simulink model "PWM_IM"  (Simulink 7.3)
settings: Solver=ode45  StartTime=0.0  StopTime=.5  RelTol=1e-3
libraries: powerlib x9
settings Model: Creator=Debmalya Mukherjee  LastModifiedBy=Debmalya Mukherjee

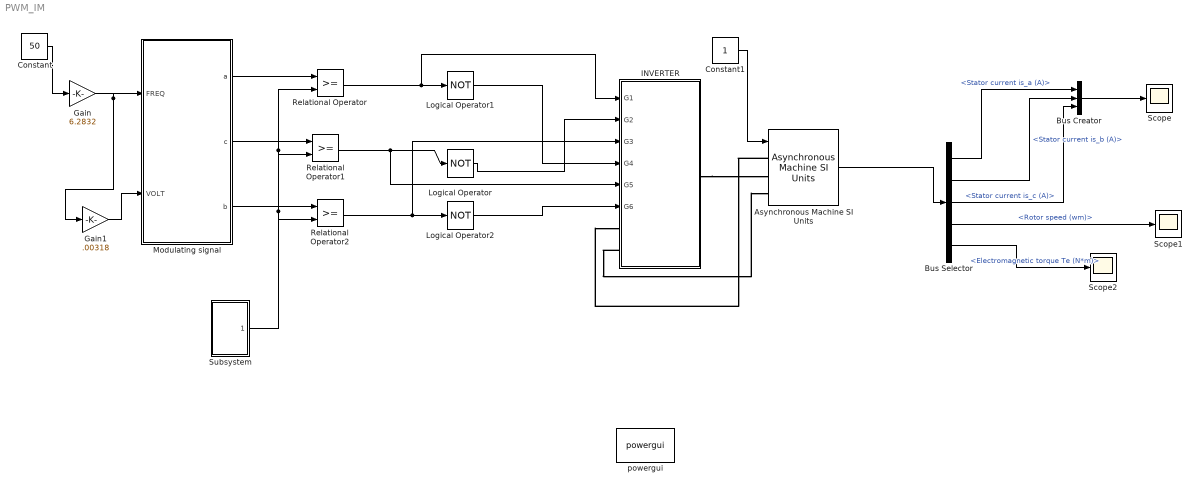
== system PWM_IM ==
  Asynchronous Machine SI Units : powerlib/Machines/Asynchronous Machine SI Units  DialogController=POWERSYS.PowerSysDialog  SystemSampleTime=-1  PresetModel=No  MechanicalLoad=Torque Tm  ShowDetailedParameters=on  RotorType=Squirrel-cage  ReferenceFrame=Rotor  NominalParameters=[10422.6 415 50 ]  Stator=[1.09 .006]  Rotor=[1.09 .006]  Lm=.072  Mechanical=[.1 .03 2]  PolePairs=2  InitialConditions=[1 0 0 0 0 0 0 0]  Units=SI  LoadFlowParameters=1492000  SimulateSaturation=off  Saturation=[14.03593122, 27.81365428, 53.79336849, 72.68890987, 97.98006896, 148.6815601, 215.7428561, 302.9841135, 428.7778367 ; 230, 322, 414, 460, 506, 552, 598, 644, 690]  TsPowergui=0  TsBlock=-1  IterativeModel=Forward Euler
  Bus Creator : BusCreator  Inputs=3
  Bus Selector : BusSelector  OutputSignals=Stator measurements.Stator current is_a (A),Stator measurements.Stator current is_b (A),Stator measurements.Stator current is_c (A),Mechanical.Rotor speed (wm),Mechanical.Electromagnetic torque Te (N*m)
  Constant : Constant  Value=50  OutDataType=fixdt(1, 16)  OutScaling=2^0
  Constant1 : Constant  OutDataType=fixdt(1, 16)  OutScaling=2^0
  Gain : Gain  Gain=6.2832  ParameterDataType=fixdt(1, 16)  ParameterScaling=2^0  OutDataType=fixdt(1, 16)  OutScaling=2^0
  Gain1 : Gain  Gain=.00318  ParameterDataType=fixdt(1, 16)  ParameterScaling=2^0  OutDataType=fixdt(1, 16)  OutScaling=2^0
  INVERTER : Subsystem
  Logical Operator : Logic  Operator=NOT  AllPortsSameDT=off  OutDataTypeMode=boolean  LogicDataType=fixdt(0, 8)  OutDataTypeStr=boolean
  Logical Operator1 : Logic  Operator=NOT  AllPortsSameDT=off  OutDataTypeMode=boolean  LogicDataType=fixdt(0, 8)  OutDataTypeStr=boolean
  Logical Operator2 : Logic  Operator=NOT  AllPortsSameDT=off  OutDataTypeMode=boolean  LogicDataType=fixdt(0, 8)  OutDataTypeStr=boolean
  Modulating signal : Subsystem
  Relational Operator : RelationalOperator  LogicOutDataTypeMode=boolean  LogicDataType=fixdt(0, 8)  OutDataTypeStr=boolean
  Relational Operator1 : RelationalOperator  LogicOutDataTypeMode=boolean  LogicDataType=fixdt(0, 8)  OutDataTypeStr=boolean
  Relational Operator2 : RelationalOperator  LogicOutDataTypeMode=boolean  LogicDataType=fixdt(0, 8)  OutDataTypeStr=boolean
  Scope : Scope
      settings: TimeRange=0.0291187739463602  YMin=-100  YMax=150
  Scope1 : Scope
  Scope2 : Scope
      settings: SaveName=ScopeData2
  Subsystem : Subsystem
  powergui : powerlib/powergui  Priority=1  SystemSampleTime=-1  SimulationMode=Continuous  SampleTime=50e-6  frequency=60  SPID=off  DisableSnubberDevices=off  DisableRonSwitches=off  DisableVfSwitches=off  SwTol=0  Interpol=off  frequencyindice=50  echomessages=off  HookPort=off  DisplayEquations=off  FunctionMessages=off  EnableUseOfTLC=off  x0status=blocks  RestoreLinks=warning  Frange=[0:2:500]  Ylog=off  Xlog=on  ShowGrid=off  save=off  variable=ZData  ZoomFFT=on  StartTime=0.0  cycles=1  DisplayStyle=1  fundamental=60  FreqAxis=off  MaxFrequency=1000  frequencyindicesteady=1  RmsSteady=1  display=off  Ts=0  methode=off
  wires:
  Constant/1 -> Gain/1
  Gain/1 -> Gain1/1, Modulating signal/1(FREQ)
  Gain1/1 -> Modulating signal/2(VOLT)
  Constant1/1 -> Asynchronous Machine SI Units/1
  Subsystem/1(Carrier) -> Relational Operator2/2, Relational Operator/2, Relational Operator1/2
  Modulating signal/1(a) -> Relational Operator/1
  Modulating signal/2(c) -> Relational Operator1/1
  Modulating signal/3(b) -> Relational Operator2/1
  Relational Operator/1 -> Logical Operator1/1, INVERTER/1(G1)
  Logical Operator1/1 -> INVERTER/4(G4)
  Relational Operator2/1 -> Logical Operator2/1, INVERTER/3(G3)
  Logical Operator2/1 -> INVERTER/6(G6)
  Relational Operator1/1 -> Logical Operator/1, INVERTER/5(G5)
  Logical Operator/1 -> INVERTER/2(G2)
  Asynchronous Machine SI Units/1 -> Bus Selector/1
  Bus Selector/1 -> Bus Creator/1  "<Stator current is_a (A)>"
  Bus Selector/2 -> Bus Creator/2  "<Stator current is_b (A)>"
  Bus Selector/3 -> Bus Creator/3  "<Stator current is_c (A)>"
  Bus Creator/1 -> Scope/1
  Bus Selector/4 -> Scope1/1  "<Rotor speed (wm)>"
  Bus Selector/5 -> Scope2/1  "<Electromagnetic torque Te (N*m)>"
  connections:
  INVERTER/RConn1 -- Asynchronous Machine SI Units/LConn2
  INVERTER/LConn2 -- Asynchronous Machine SI Units/LConn3
  Asynchronous Machine SI Units/LConn1 -- INVERTER/LConn1

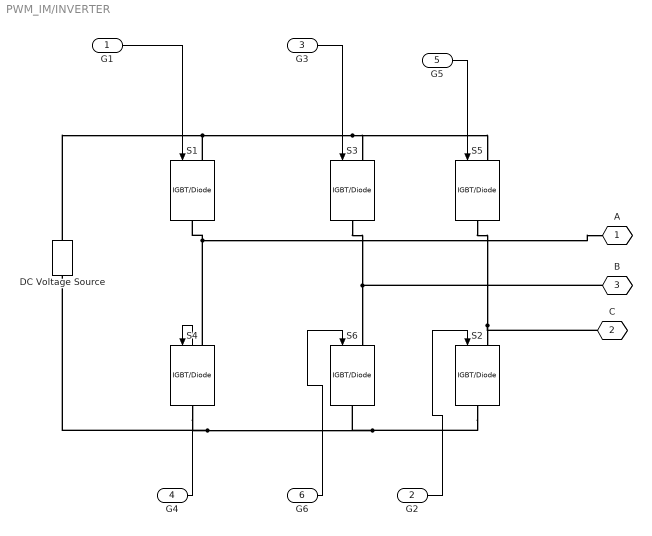
== system PWM_IM/INVERTER ==
  G1 : Inport  OutDataType=fixdt(1, 16)  OutScaling=2^0
  G2 : Inport  Port=2  OutDataType=fixdt(1, 16)  OutScaling=2^0
  G3 : Inport  Port=3  OutDataType=fixdt(1, 16)  OutScaling=2^0
  G4 : Inport  Port=4  OutDataType=fixdt(1, 16)  OutScaling=2^0
  G5 : Inport  Port=5  OutDataType=fixdt(1, 16)  OutScaling=2^0
  G6 : Inport  Port=6  OutDataType=fixdt(1, 16)  OutScaling=2^0
  DC Voltage Source : powerlib/Electrical Sources/DC Voltage Source  DialogController=POWERSYS.PowerSysDialog  SystemSampleTime=-1  Amplitude=600  Measurements=None
  S{1..6} (6 alike) : powerlib/Power Electronics/IGBT//Diode  DialogController=POWERSYS.PowerSysDialog  SystemSampleTime=-1  Ron=1e-3  Rs=1e5  Cs=inf  Measurements=off
  A : PMIOPort  Tag=PMCPort  Port=1  Side=Left
  C : PMIOPort  Tag=PMCPort  Port=2  Side=Left
  B : PMIOPort  Tag=PMCPort  Port=3  Side=Right
  wires:
  G1/1 -> S1/1
  G2/1 -> S2/1
  G3/1 -> S3/1
  G4/1 -> S4/1
  G5/1 -> S5/1
  G6/1 -> S6/1
  connections:
  S2/RConn1 -- S6/RConn1 -- DC Voltage Source/LConn1 -- S4/RConn1
  DC Voltage Source/RConn1 -- S1/LConn1 -- S3/LConn1 -- S5/LConn1
  A/RConn1 -- S4/LConn1 -- S1/RConn1
  C/RConn1 -- S5/RConn1 -- S2/LConn1
  S3/RConn1 -- S6/LConn1 -- B/RConn1

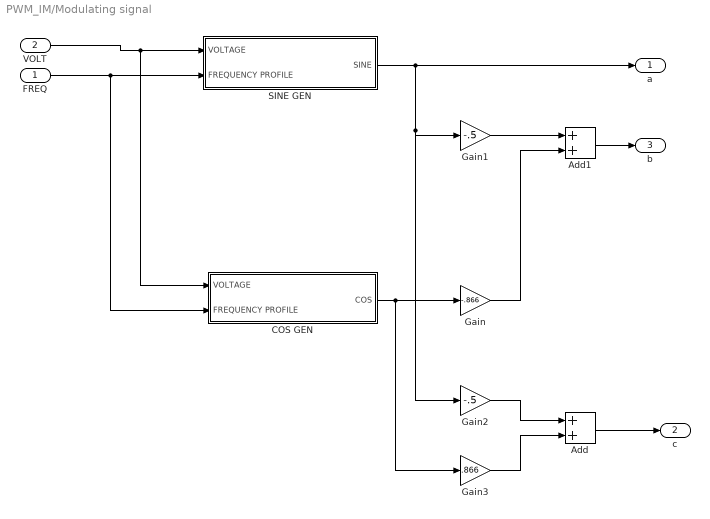
== system PWM_IM/Modulating signal ==
  FREQ : Inport  OutDataType=fixdt(1, 16)  OutScaling=2^0
  VOLT : Inport  Port=2  OutDataType=fixdt(1, 16)  OutScaling=2^0
  Add : Sum  OutDataType=fixdt(1, 16)  OutScaling=2^-10
  Add1 : Sum  OutDataType=fixdt(1, 16)  OutScaling=2^-10
  COS GEN : Subsystem
  Gain : Gain  Gain=-.866  ParameterDataType=fixdt(1, 16)  ParameterScaling=2^0  OutDataType=fixdt(1, 16)  OutScaling=2^0
  Gain1 : Gain  Gain=-.5  ParameterDataType=fixdt(1, 16)  ParameterScaling=2^0  OutDataType=fixdt(1, 16)  OutScaling=2^0
  Gain2 : Gain  Gain=-.5  ParameterDataType=fixdt(1, 16)  ParameterScaling=2^0  OutDataType=fixdt(1, 16)  OutScaling=2^0
  Gain3 : Gain  Gain=.866  ParameterDataType=fixdt(1, 16)  ParameterScaling=2^0  OutDataType=fixdt(1, 16)  OutScaling=2^0
  SINE GEN : Subsystem
  a : Outport  OutDataType=fixdt(1, 16)  OutScaling=2^0
  c : Outport  Port=2  OutDataType=fixdt(1, 16)  OutScaling=2^0
  b : Outport  Port=3  OutDataType=fixdt(1, 16)  OutScaling=2^0
  wires:
  FREQ/1 -> SINE GEN/2(FREQUENCY PROFILE), COS GEN/2(FREQUENCY PROFILE)
  VOLT/1 -> SINE GEN/1(VOLTAGE), COS GEN/1(VOLTAGE)
  SINE GEN/1(SINE) -> a/1, Gain1/1, Gain2/1
  Gain1/1 -> Add1/1
  Add1/1 -> b/1
  COS GEN/1(COS) -> Gain/1, Gain3/1
  Gain/1 -> Add1/2
  Gain3/1 -> Add/2
  Gain2/1 -> Add/1
  Add/1 -> c/1

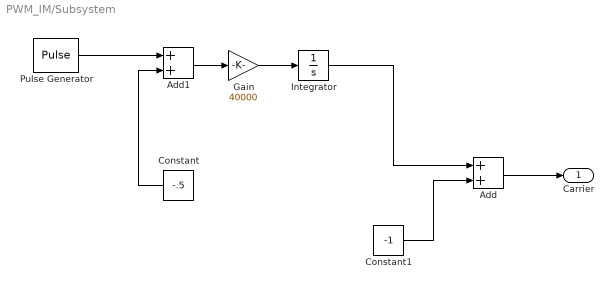
== system PWM_IM/Subsystem ==
  Add : Sum  OutDataType=fixdt(1, 16)  OutScaling=2^-10
  Add1 : Sum  OutDataType=fixdt(1, 16)  OutScaling=2^-10
  Constant : Constant  Value=-.5  OutDataType=fixdt(1, 16)  OutScaling=2^0
  Constant1 : Constant  Value=-1  OutDataType=fixdt(1, 16)  OutScaling=2^0
  Gain : Gain  Gain=40000  ParameterDataType=fixdt(1, 16)  ParameterScaling=2^0  OutDataType=fixdt(1, 16)  OutScaling=2^0
  Integrator : Integrator
  Pulse Generator : DiscretePulseGenerator  PulseType=Time based  Amplitude=1  Period=.0002  PulseWidth=50  PhaseDelay=0  SampleTime=1
  Carrier : Outport  OutDataType=fixdt(1, 16)  OutScaling=2^0
  wires:
  Pulse Generator/1 -> Add1/1
  Constant/1 -> Add1/2
  Add1/1 -> Gain/1
  Gain/1 -> Integrator/1
  Add/1 -> Carrier/1
  Constant1/1 -> Add/2
  Integrator/1 -> Add/1

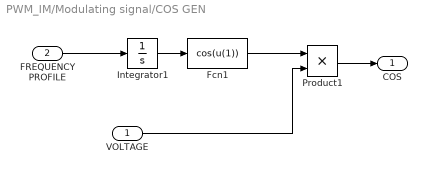
== system PWM_IM/Modulating signal/COS GEN ==
  VOLTAGE : Inport  OutDataType=fixdt(1, 16)  OutScaling=2^0
  FREQUENCY PROFILE : Inport  Port=2  OutDataType=fixdt(1, 16)  OutScaling=2^0
  Fcn1 : Fcn  Expr=cos(u(1))
  Integrator1 : Integrator
  Product1 : Product  OutDataType=fixdt(1, 16)  OutScaling=2^0  RndMeth=Zero
  COS : Outport  OutDataType=fixdt(1, 16)  OutScaling=2^0
  wires:
  FREQUENCY PROFILE/1 -> Integrator1/1
  Integrator1/1 -> Fcn1/1
  Fcn1/1 -> Product1/1
  VOLTAGE/1 -> Product1/2
  Product1/1 -> COS/1

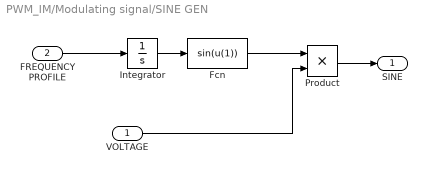
== system PWM_IM/Modulating signal/SINE GEN ==
  VOLTAGE : Inport  OutDataType=fixdt(1, 16)  OutScaling=2^0
  FREQUENCY PROFILE : Inport  Port=2  OutDataType=fixdt(1, 16)  OutScaling=2^0
  Fcn : Fcn  Expr=sin(u(1))
  Integrator : Integrator
  Product : Product  OutDataType=fixdt(1, 16)  OutScaling=2^0  RndMeth=Zero
  SINE : Outport  OutDataType=fixdt(1, 16)  OutScaling=2^0
  wires:
  FREQUENCY PROFILE/1 -> Integrator/1
  Integrator/1 -> Fcn/1
  Fcn/1 -> Product/1
  VOLTAGE/1 -> Product/2
  Product/1 -> SINE/1
